simulink model "ThrusterSolver"  (R2022b)
settings: Solver=VariableStepAuto  StartTime=0.0  StopTime=10.0  RelTol=1e-3
undefined symbols (not defined in the file or in its folder): importedData
settings Model: Creator=hollis  LastModifiedBy=hollis

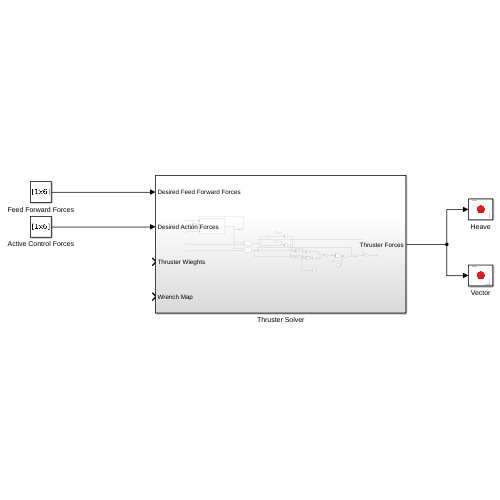
[thumbnail: Simulink's stored preview of the top-level diagram]
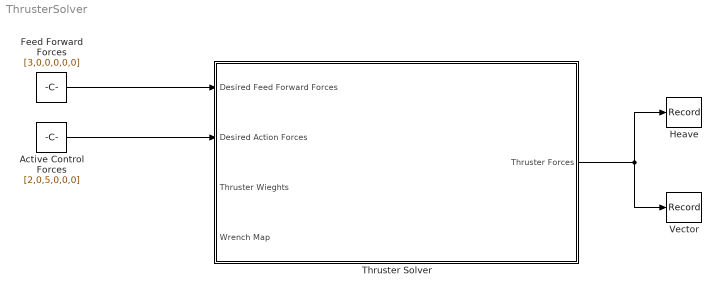
== system ThrusterSolver ==
  Active Control Forces : Constant  Value=[2,0,5,0,0,0]
  Feed Forward Forces : Constant  Value=[3,0,0,0,0,0]
  Heave : Record  FileSettingsInternal="{\"entries\":[{\"content\":{\"excelSettings\":{\"content\":{},\"type\":\"Streamout.ExcelSettings\"}},\"type\":\"Streamout.FileSettingStorage\",\"uuid\":\"8f45ba7d-dfe0-464b-af19-a81f3c0c178c\"}],\"packageUris\":[\"http://schema.mathworks.com/mf0/streamout_blocks/R2020a\"],\"version\":\"1.0\"}"  Layout=[1 1]  SignalsInternal="{\"entries\":[{\"content\":{\"signals\":[{\"content\":{\"blockPath\":[\"ThrusterSolver/Heave\"],\"channel\":[],\"dimensions\":[8],\"domain\":\"ThrusterSolver/Heave\",\"hasChildren\":true,\"lineColor\":\"#7e2f8e\",\"plots\":[],\"port\":1,\"sid\":[],\"signalID\":133,\"signalName\":\"Subsystem\"},\"type\":\"RecordBlkView.Signal\",\"uuid\":\"bb934f69-8ba5-4c6f-b336-481211658a67\"},{\"content\":{\"blockPath\":[\"ThrusterSolver/Heave\"],\"channel\":[1],\"dimensions\":[8],\"domain\":\"ThrusterSolver/Heave\",\"lineColor\":\"#d95319\",\"parentID\":133,\"plots\":[],\"port\":1,\"sid\":[],\"signalID\":134,\"signalName\":\"Subsystem\"},\"type\":\"RecordBlkView.Signal\",\"uuid\":\"ba37456c-9e7d-4cfd-8940-3389acad7e3b\"},{\"content\":{\"blockPath\":[\"ThrusterSolver/Heave\"],\"channel\":[2],\"dimensions\":[8],\"domain\":\"ThrusterSolver/Heave\",\"lineColor\":\"#77ac30\",\"parentID\":133,\"plots\":[],\"port\":1,\"sid\":[],\"signalID\":135,\"signalName\":\"Subsystem\"},\"type\":\"RecordBlkView.Signal\",\"uuid\":\"e6bf9be1-7c06-462e-a128-53d6add41167\"},{\"content\":{\"blockPath\":[\"ThrusterSolver/Heave\"],\"channel\":[3],\"dimensions\":[8],\"domain\":\"ThrusterSolver/Heave\",\"lineColor\":\"#4dbeee\",\"parentID\":133,\"plots\":[],\"port\":1,\"sid\":[],\"signalID\":136,\"signalName\":\"Subsystem\"},\"type\":\"RecordBlkView.Signal\",\"uuid\":\"847de211-840b-4a19-9506-b22bcdaf5a6c\"},{\"content\":{\"blockPath\":[\"ThrusterSolver/Heave\"],\"channel\":[4],\"dimensions\":[8],\"domain\":\"ThrusterSolver/Heave\",\"lineColor\":\"#a2142f\",\"parentID\":133,\"plots\":[],\"port\":1,\"sid\":[],\"signalID\":137,\"signalName\":\"Subsystem\"},\"type\":\"RecordBlkView.Signal\",\"uuid\":\"e25e0dd7-5f4a-4449-b0a9-04ded1912196\"},{\"content\":{\"blockPath\":[\"ThrusterSolver/Heave\"],\"channel\":[5],\"dimensions\":[8],\"domain\":\"ThrusterSolver/Heave\",\"lineColor\":\"#139fff\",\"parentID\":133,\"plots\":[1],\"port\":1,\"sid\":[],\"signalID\":138,\"signalName\":\"Subsystem\"},\"type\":\"RecordBlkView.Signal\",\"uuid\":\"fc1388c6-beb1-4a56-90d3-5bb20ffb0099\"},{\"content\":{\"blockPath\":[\"ThrusterSolver/Heave\"],\"channel\":[6],\"dimensions\":[8],\"domain\":\"ThrusterSolver/Heave\",\"lineColor\":\"#ff6929\",\"parentID\":133,\"plots\":[1],\"port\":1,\"sid\":[],\"signalID\":139,\"signalName\":\"Subsystem\"},\"type\":\"RecordBlkView.Signal\",\"uuid\":\"8a02418c-d2a3-4184-9128-7424c43d89d4\"},{\"content\":{\"blockPath\":[\"ThrusterSolver/Heave\"],\"channel\":[7],\"dimensions\":[8],\"domain\":\"ThrusterSolver/Heave\",\"lineColor\":\"#b746ff\",\"parentID\":133,\"plots\":[1],\"port\":1,\"sid\":[],\"signalID\":140,\"signalName\":\"Subsystem\"},\"type\":\"RecordBlkView.Signal\",\"uuid\":\"89adbacf-e049-48bb-b1cb-acc1ac2cd20d\"},{\"content\":{\"blockPath\":[\"ThrusterSolver/Heave\"],\"channel\":[8],\"dimensions\":[8],\"domain\":\"ThrusterSolver/Heave\",\"lineColor\":\"#64d413\",\"parentID\":133,\"plots\":[1],\"port\":1,\"sid\":[],\"signalID\":141,\"signalName\":\"Subsystem\"},\"type\":\"RecordBlkView.Signal\",\"uuid\":\"2bec8fd7-ab92-49ea-9335-61ac1474049a\"}]},\"type\":\"RecordBlkView.InputSignals\",\"uuid\":\"aebfee86-83ed-410a-a850-a31a572cfaaf\"}],\"packageUris\":[\"http://schema.mathworks.com/mf0/streamout_blocks/R2020a\"],\"version\":\"1.0\"}"  VisualizationBindings="{\"sparklinesplugin\":{\"info\":[{\"bindingParametersList\":[],\"subplotID\":1}]}}"
  Thruster Solver : Subsystem
  Vector : Record  FileSettingsInternal="{\"entries\":[{\"content\":{\"excelSettings\":{\"content\":{},\"type\":\"Streamout.ExcelSettings\"}},\"type\":\"Streamout.FileSettingStorage\",\"uuid\":\"61bd1469-b984-4ec0-b365-8bb8eebf11d9\"}],\"packageUris\":[\"http://schema.mathworks.com/mf0/streamout_blocks/R2020a\"],\"version\":\"1.0\"}"  Layout=[1 1]  SignalsInternal="{\"entries\":[{\"content\":{\"signals\":[{\"content\":{\"blockPath\":[\"ThrusterSolver/Vector\"],\"channel\":[],\"dimensions\":[8],\"domain\":\"ThrusterSolver/Vector\",\"hasChildren\":true,\"lineColor\":\"#4dbeee\",\"plots\":[],\"port\":1,\"sid\":[],\"signalID\":112,\"signalName\":\"Subsystem\"},\"type\":\"RecordBlkView.Signal\",\"uuid\":\"6b9398d0-8540-41e8-b1b9-14589be4269f\"},{\"content\":{\"blockPath\":[\"ThrusterSolver/Vector\"],\"channel\":[1],\"dimensions\":[8],\"domain\":\"ThrusterSolver/Vector\",\"lineColor\":\"#7e2f8e\",\"parentID\":112,\"plots\":[1],\"port\":1,\"sid\":[],\"signalID\":113,\"signalName\":\"Subsystem\"},\"type\":\"RecordBlkView.Signal\",\"uuid\":\"3a09ebe4-e56c-4447-924f-3716de9a2e02\"},{\"content\":{\"blockPath\":[\"ThrusterSolver/Vector\"],\"channel\":[2],\"dimensions\":[8],\"domain\":\"ThrusterSolver/Vector\",\"lineColor\":\"#ff6929\",\"parentID\":112,\"plots\":[1],\"port\":1,\"sid\":[],\"signalID\":114,\"signalName\":\"Subsystem\"},\"type\":\"RecordBlkView.Signal\",\"uuid\":\"b37158be-b5f8-4aa4-bad9-f8b7a425c53c\"},{\"content\":{\"blockPath\":[\"ThrusterSolver/Vector\"],\"channel\":[3],\"dimensions\":[8],\"domain\":\"ThrusterSolver/Vector\",\"lineColor\":\"#b746ff\",\"parentID\":112,\"plots\":[1],\"port\":1,\"sid\":[],\"signalID\":115,\"signalName\":\"Subsystem\"},\"type\":\"RecordBlkView.Signal\",\"uuid\":\"b841f9e1-2560-4fcd-b4d5-43c307cd4cbb\"},{\"content\":{\"blockPath\":[\"ThrusterSolver/Vector\"],\"channel\":[4],\"dimensions\":[8],\"domain\":\"ThrusterSolver/Vector\",\"lineColor\":\"#64d413\",\"parentID\":112,\"plots\":[1],\"port\":1,\"sid\":[],\"signalID\":116,\"signalName\":\"Subsystem\"},\"type\":\"RecordBlkView.Signal\",\"uuid\":\"6da6b886-ef72-4c87-a7de-a92b0cdd6865\"},{\"content\":{\"blockPath\":[\"ThrusterSolver/Vector\"],\"channel\":[5],\"dimensions\":[8],\"domain\":\"ThrusterSolver/Vector\",\"lineColor\":\"#ff13a6\",\"parentID\":112,\"plots\":[],\"port\":1,\"sid\":[],\"signalID\":117,\"signalName\":\"Subsystem\"},\"type\":\"RecordBlkView.Signal\",\"uuid\":\"a151a52e-573b-451c-8b2d-18d3b6d3bde0\"},{\"content\":{\"blockPath\":[\"ThrusterSolver/Vector\"],\"channel\":[6],\"dimensions\":[8],\"domain\":\"ThrusterSolver/Vector\",\"lineColor\":\"#fe330a\",\"parentID\":112,\"plots\":[],\"port\":1,\"sid\":[],\"signalID\":118,\"signalName\":\"Subsystem\"},\"type\":\"RecordBlkView.Signal\",\"uuid\":\"4741ba58-157e-4e86-8178-ceb78517568b\"},{\"content\":{\"blockPath\":[\"ThrusterSolver/Vector\"],\"channel\":[7],\"dimensions\":[8],\"domain\":\"ThrusterSolver/Vector\",\"lineColor\":\"#22b573\",\"parentID\":112,\"plots\":[],\"port\":1,\"sid\":[],\"signalID\":119,\"signalName\":\"Subsystem\"},\"type\":\"RecordBlkView.Signal\",\"uuid\":\"d6f6f60e-9e6d-4319-ae7e-a95665305af3\"},{\"content\":{\"blockPath\":[\"ThrusterSolver/Vector\"],\"channel\":[8],\"dimensions\":[8],\"domain\":\"ThrusterSolver/Vector\",\"lineColor\":\"#0072bd\",\"parentID\":112,\"plots\":[],\"port\":1,\"sid\":[],\"signalID\":120,\"signalName\":\"Subsystem\"},\"type\":\"RecordBlkView.Signal\",\"uuid\":\"0cdf5d76-c3db-41e2-ab67-0fe1c619c1d0\"}]},\"type\":\"RecordBlkView.InputSignals\",\"uuid\":\"7d5e8d02-647d-4a9c-87e5-e902a66a40bd\"}],\"packageUris\":[\"http://schema.mathworks.com/mf0/streamout_blocks/R2020a\"],\"version\":\"1.0\"}"  VisualizationBindings="{\"sparklinesplugin\":{\"info\":[{\"bindingParametersList\":[],\"subplotID\":1}]}}"
  wires:
  Feed Forward Forces/1 -> Thruster Solver/1(Desired Feed Forward Forces)
  Active Control Forces/1 -> Thruster Solver/2(Desired Action Forces)
  Thruster Solver/1(Thruster Forces) -> Vector/1, Heave/1

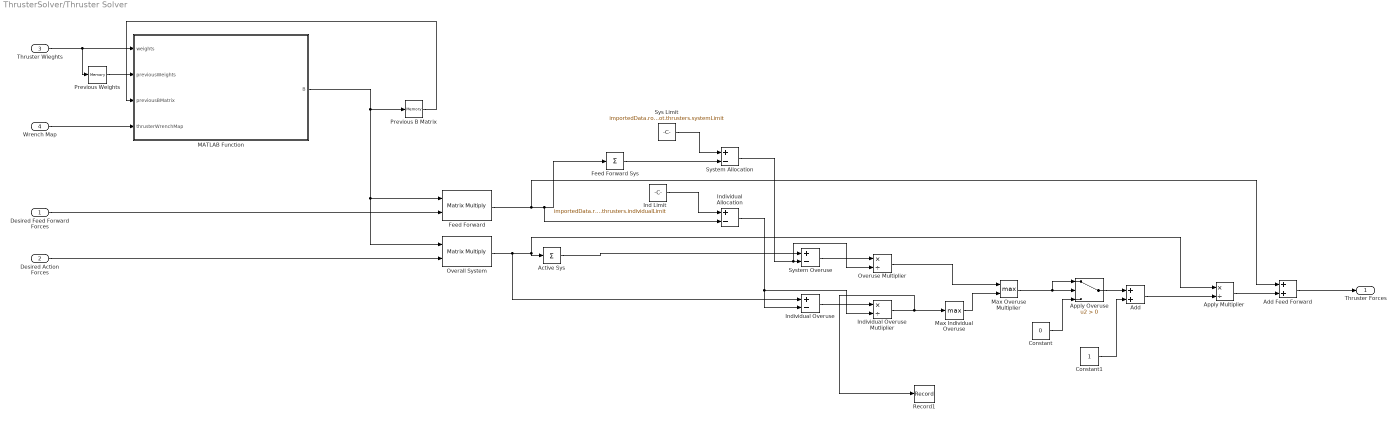
== system ThrusterSolver/Thruster Solver ==
  Desired Feed Forward Forces : Inport
  Desired Action Forces : Inport  Port=2
  Thruster Wieghts : Inport  Port=3
  Wrench Map : Inport  Port=4
  Active Sys : Sum  Inputs=+
  Add : Sum
  Add Feed Forward : Sum
  Apply Multiplier : Product  Inputs=*/
  Apply Overuse : Switch  Criteria=u2 > Threshold  SaturateOnIntegerOverflow=off  InputSameDT=off
  Constant : Constant  Value=0
  Constant1 : Constant
  "Feed Forward " : Product  Multiplication=Matrix(*)
  Feed Forward Sys : Sum  Inputs=+
  Ind Limit : Constant  Value=importedData.robot.thrusters.individualLimit  VectorParams1D=off
  Individual Allocation : Sum  Inputs=+-
  Individual Overuse : Sum  Inputs=+-
  Individual Overuse Mutliplier : Product  Inputs=*/
  MATLAB Function : MATLAB Function  TreatAsAtomicUnit=on
  Max Individual Overuse : MinMax  Function=max
  Max Overuse Multiplier : MinMax  Function=max  Inputs=2
  Overall System : Product  Multiplication=Matrix(*)
  Overuse Multiplier : Product  Inputs=*/
  Previous B Matrix : Memory
  Previous Weights : Memory
  Record1 : Record  FileSettingsInternal="{\"entries\":[{\"content\":{\"excelSettings\":{\"content\":{},\"type\":\"Streamout.ExcelSettings\"}},\"type\":\"Streamout.FileSettingStorage\",\"uuid\":\"0a4dd645-a325-4954-be18-2a7cdcc32f58\"}],\"packageUris\":[\"http://schema.mathworks.com/mf0/streamout_blocks/R2020a\"],\"version\":\"1.0\"}"  Layout=[1 1]  SignalsInternal="{\"entries\":[{\"content\":{\"signals\":[{\"content\":{\"blockPath\":[\"ThrusterSolver/Subsystem/Record1\"],\"channel\":[],\"dimensions\":[8],\"domain\":\"ThrusterSolver/Subsystem/Record1\",\"hasChildren\":true,\"lineColor\":\"#139fff\",\"plots\":[],\"port\":1,\"sid\":[],\"signalID\":98,\"signalName\":\"Individual Overuse Mutliplier\"},\"type\":\"RecordBlkView.Signal\",\"uuid\":\"977c9520-5e4b-4bf1-90ea-e70d73eebe3d\"},{\"content\":{\"blockPath\":[\"ThrusterSolver/Subsystem/Record1\"],\"channel\":[1],\"dimensions\":[8],\"domain\":\"ThrusterSolver/Subsystem/Record1\",\"lineColor\":\"#7e2f8e\",\"parentID\":98,\"plots\":[],\"port\":1,\"sid\":[],\"signalID\":99,\"signalName\":\"Individual Overuse Mutliplier\"},\"type\":\"RecordBlkView.Signal\",\"uuid\":\"8b9d17b5-4a68-493b-8ae6-5e71ec768666\"}]},\"type\":\"RecordBlkView.InputSignals\",\"uuid\":\"cbd002b3-ba51-4923-ab8b-32ff9cbc01c8\"}],\"packageUris\":[\"http://schema.mathworks.com/mf0/streamout_blocks/R2020a\"],\"version\":\"1.0\"}"  VisualizationBindings="{\"sparklinesplugin\":{\"info\":[{\"bindingParametersList\":[],\"subplotID\":1}]}}"
  Sys Limit : Constant  Value=importedData.robot.thrusters.systemLimit
  System Allocation : Sum  Inputs=+-
  System Overuse : Sum  Inputs=+-
  Thruster Forces : Outport
  wires:
  Constant/1 -> Apply Overuse/3
  Feed Forward Sys/1 -> System Allocation/2
  Individual Overuse/1 -> Individual Overuse Mutliplier/1
  Individual Allocation/1 -> Individual Overuse Mutliplier/2, Individual Overuse/2
  Overall System/1 -> Individual Overuse/1, Apply Multiplier/1, Active Sys/1
  Max Overuse Multiplier/1 -> Apply Overuse/1, Apply Overuse/2
  Desired Feed Forward Forces/1 -> "Feed Forward "/2
  System Overuse/1 -> Overuse Multiplier/1
  Active Sys/1 -> System Overuse/1
  Apply Multiplier/1 -> Add Feed Forward/2
  Overuse Multiplier/1 -> Max Overuse Multiplier/1
  Max Individual Overuse/1 -> Max Overuse Multiplier/2
  System Allocation/1 -> Overuse Multiplier/2, System Overuse/2
  Ind Limit/1 -> Individual Allocation/1
  Desired Action Forces/1 -> Overall System/2
  "Feed Forward "/1 -> Add Feed Forward/1, Individual Allocation/2, Feed Forward Sys/1
  Constant1/1 -> Add/2
  Individual Overuse Mutliplier/1 -> Record1/1, Max Individual Overuse/1
  Sys Limit/1 -> System Allocation/1
  Apply Overuse/1 -> Add/1
  Add/1 -> Apply Multiplier/2
  Add Feed Forward/1 -> Thruster Forces/1
  MATLAB Function/1(B) -> Previous B Matrix/1, Overall System/1, "Feed Forward "/1
  Previous B Matrix/1 -> MATLAB Function/3(previousBMatrix)
  Wrench Map/1 -> MATLAB Function/4(thrusterWrenchMap)
  Thruster Wieghts/1 -> MATLAB Function/1(weights), Previous Weights/1
  Previous Weights/1 -> MATLAB Function/2(previousWeights)

== matlab function ThrusterSolver/Thruster Solver/MATLAB Function ==
  data: weights input; B output; previousWeights input; previousBMatrix input; thrusterWrenchMap input
function B = generateBMatrix(weights, previousWeights, previousBMatrix, thrusterWrenchMap)

    if(isequal(weights, previousWeights))
        %if the weights are the same, just send the previous B matrix
        B = previousBMatrix;
        return
    end

    %if new weights, calculate the a new b matrix
    weightsMatrix = diag(weights);
    B = inv(weightsMatrix) * (thrusterWrenchMap) * inv((transpose(thrusterWrenchMap) * inv(weightsMatrix) * (thrusterWrenchMap)));
